simulink model "single_camera_xy_tracking_base_cv_kf"  (R2025b)
settings: Solver=FixedStepDiscrete  StartTime=0  StopTime=T_end  FixedStep=Ts  RelTol=1e-3
InitFcn:
  | config_dir=fullfile(fileparts(get_param(bdroot,'FileName')),'..','config');
  | addpath(config_dir);
  | init_single_camera_xy_tracking_base_cv_kf;
values from neighbouring files (symbols this model uses):
  Kpx = parameters(3)    [build_single_camera_joint_velocity_direct.m]    (also in build_single_camera_joint_velocity_direct1.m)
  Kpy = parameters(4);",  "k_ff=parameters(5)    [build_single_camera_joint_velocity_direct.m]    (also in build_single_camera_joint_velocity_direct1.m)
  Z_hat = parameters(2)    [build_single_camera_joint_velocity_direct.m]    (also in build_single_camera_joint_velocity_direct1.m)
undefined symbols (not defined in the file or in its folder): a_xy_max, controller_enable, data, data_SL_Info, enable_ekf_feedforward, enable_proportional, ff_ramp_time, joint_buffer_capacity, joint_state_timeout_sec, k_ff, measurement_reset_timeout, nis_position_threshold, nis_velocity_threshold, P0, pending_visual_capacity, Q_kf, R_position, R_velocity, required_valid_frames, sync_allow_extrapolation, sync_clock_reset_threshold_sec, sync_max_bracket_span_sec, sync_max_visual_wait_sec, sync_required_for_control, target_timeout_sec, Ts, v_xy_max
libraries: ros2lib x5, robotmaniplib x2
(part 2 of 2)

== matlab function single_camera_xy_tracking_base_cv_kf/Joint State ROS2 Subscriber/Joint Source Timestamp ==
  data: sec input size=1; joint_source_stamp output size=1; nsec input size=1; joint_source_stamp_valid output size=1
function [joint_source_stamp,joint_source_stamp_valid] = fcn(sec,nsec)
%#codegen
% 将 JointState Header 的 sec/nanosec 校验并转换为 ROS 源时间。
joint_source_stamp=0;
joint_source_stamp_valid=0;
sec=double(sec);
nsec=double(nsec);
ok=isfinite(sec)&&sec>=0&&sec==floor(sec)&& ...
    isfinite(nsec)&&nsec>=0&&nsec<1e9&&nsec==floor(nsec);
if ~ok
    return
end
joint_source_stamp=sec+1e-9*nsec;
joint_source_stamp_valid=double(isfinite(joint_source_stamp)&&joint_source_stamp>0);
end

== matlab function single_camera_xy_tracking_base_cv_kf/Visual Joint Time Alignment/Align JointState to Visual Time ==
  data: position_C input size=[2 1]; aligned_position_C output size=[2 1]; relative_velocity_C input size=[2 1]; position_valid input size=1; velocity_valid input size=1; visual_source_stamp input size=1; visual_source_stamp_valid input size=1; visual_message_is_new input size=1; joint_position input size=[7 1]; joint_velocity input size=[7 1]; joint_count input size=1; joint_age input size=1; joint_source_stamp input size=1; joint_source_stamp_valid input size=1; joint_message_is_new input size=1; sim_time input size=1; parameters input size=[8 1]; aligned_relative_velocity_C output size=[2 1]; aligned_q output size=[7 1]; aligned_qdot output size=[7 1]; aligned_visual_stamp output size=1; aligned_joint_stamp_0 output size=1; aligned_joint_stamp_1 output size=1; sync_alpha output size=1; sync_bracket_span output size=1; sync_wait_time output size=1; sync_valid output size=1; aligned_measurement_is_new output size=1; aligned_position_valid output size=1; aligned_velocity_valid output size=1; sync_drop_reason output size=1; joint_buffer_count output size=1; pending_visual_count output size=1; joint_out_of_order_drop_count output size=1; visual_sync_drop_count output size=1; clock_reset_count output size=1; sync_reset_required output size=1
function [aligned_position_C,aligned_relative_velocity_C,aligned_q, ...
    aligned_qdot,aligned_visual_stamp,aligned_joint_stamp_0, ...
    aligned_joint_stamp_1,sync_alpha,sync_bracket_span,sync_wait_time, ...
    sync_valid,aligned_measurement_is_new,aligned_position_valid, ...
    aligned_velocity_valid,sync_drop_reason,joint_buffer_count, ...
    pending_visual_count,joint_out_of_order_drop_count, ...
    visual_sync_drop_count,clock_reset_count,sync_reset_required] = fcn( ...
    position_C,relative_velocity_C,position_valid,velocity_valid, ...
    visual_source_stamp,visual_source_stamp_valid,visual_message_is_new, ...
    joint_position,joint_velocity,joint_count,joint_age, ...
    joint_source_stamp,joint_source_stamp_valid,joint_message_is_new, ...
    sim_time,parameters)
%#codegen
% 缓存 JointState，并在视觉源时刻包围插值关节状态。
[aligned_position_C,aligned_relative_velocity_C,aligned_q, ...
    aligned_qdot,aligned_visual_stamp,aligned_joint_stamp_0, ...
    aligned_joint_stamp_1,sync_alpha,sync_bracket_span,sync_wait_time, ...
    sync_valid_raw,aligned_measurement_is_new_raw,aligned_position_valid_raw, ...
    aligned_velocity_valid_raw,sync_drop_reason,joint_buffer_count, ...
    pending_visual_count,joint_out_of_order_drop_count, ...
    visual_sync_drop_count,clock_reset_count,sync_reset_required_raw]= ...
    joint_visual_time_aligner_step(position_C,relative_velocity_C, ...
    position_valid,velocity_valid,visual_source_stamp, ...
    visual_source_stamp_valid,visual_message_is_new,joint_position, ...
    joint_velocity,joint_count,joint_age,joint_source_stamp, ...
    joint_source_stamp_valid,joint_message_is_new,sim_time, ...
    parameters(1),parameters(2),parameters(3),parameters(4), ...
    parameters(5),parameters(6),parameters(7),parameters(8));
sync_valid=double(sync_valid_raw);
aligned_measurement_is_new=double(aligned_measurement_is_new_raw);
aligned_position_valid=double(aligned_position_valid_raw);
aligned_velocity_valid=double(aligned_velocity_valid_raw);
sync_reset_required=double(sync_reset_required_raw);
end

== matlab function single_camera_xy_tracking_base_cv_kf/Target ROS2 Subscriber/Unpack ==
  data: data input; target_data output size=[8 1]; is_new input size=1; t input size=1; target_count output size=1; target_age output size=1
function [target_data,target_count,target_age] = fcn(data,is_new,t)
%#codegen
% 缓存带图像源时间戳的固定八元素视觉消息。
persistent last_data last_count last_time
if isempty(last_count)
    last_data=zeros(8,1);
    last_count=0;
    last_time=-1e6;
end
if is_new
    n=numel(data);
    last_data=zeros(8,1);
    for k=1:min(n,8)
        last_data(k)=double(data(k));
    end
    last_count=double(n);
    last_time=t;
end
target_data=last_data;
target_count=last_count;
target_age=max(0,t-last_time);
end

== matlab function single_camera_xy_tracking_base_cv_kf/Target Measurement Validation/Validate Timestamped Visual ==
  data: target_data input size=[8 1]; position_valid output size=1; target_count input size=1; target_age input size=1; target_timeout_sec input size=1; velocity_valid output size=1; position_C output size=[2 1]; relative_velocity_C output size=[2 1]; visual_source_stamp output size=1; visual_source_stamp_valid output size=1
function [position_valid,velocity_valid,position_C,relative_velocity_C, ...
    visual_source_stamp,visual_source_stamp_valid] = fcn( ...
    target_data,target_count,target_age,target_timeout_sec)
%#codegen
% 解析并校验带图像源时间戳的八元素视觉消息。
[position_valid_raw,velocity_valid_raw,position_C,relative_velocity_C, ...
    visual_source_stamp,visual_source_stamp_valid_raw]= ...
    parse_target_measurement(target_data,target_count,target_age, ...
    target_timeout_sec);
position_valid=double(position_valid_raw);
velocity_valid=double(velocity_valid_raw);
visual_source_stamp_valid=double(visual_source_stamp_valid_raw);
end

== matlab function single_camera_xy_tracking_base_cv_kf/Joint State ROS2 Subscriber/Unpack ==
  data: position input; joint_position output size=[7 1]; velocity input; is_new input size=1; t input size=1; joint_count output size=1; joint_velocity output size=[7 1]; joint_age output size=1
function [joint_position,joint_count,joint_velocity,joint_age] = fcn(position,velocity,is_new,t)
%#codegen
persistent last_q last_dq last_count last_time
if isempty(last_count), last_q=zeros(7,1); last_dq=zeros(7,1); last_count=0.0; last_time=-1.0e6; end
if is_new
    np=numel(position); nv=numel(velocity); last_q=zeros(7,1); last_dq=zeros(7,1);
    for k=1:min(np,7), last_q(k)=position(k); end
    for k=1:min(nv,7), last_dq(k)=velocity(k); end
    last_count=double(min(np,nv)); last_time=t;
end
joint_position=last_q; joint_count=last_count; joint_velocity=last_dq; joint_age=max(0.0,t-last_time);
end

== matlab function single_camera_xy_tracking_base_cv_kf/Measured Camera Twist in Base/Measured Twist ==
  data: J_camera_base input size=[6 7]; camera_twist_base output size=[6 1]; joint_velocity input size=[7 1]; T_camera2base input size=[4 4]; joint_motion_valid input; joint_geometry_valid input; camera_motion_valid output; T_camera2base_out output size=[4 4]
function [camera_twist_base,camera_motion_valid,T_camera2base_out] = fcn( ...
    J_camera_base,joint_velocity,T_camera2base,joint_motion_valid, ...
    joint_geometry_valid)
%#codegen
% 使用已校验的实测关节速度计算 Base 系相机 Twist。
camera_twist_base=zeros(6,1);
camera_motion_valid=false;
T_camera2base_out=zeros(4,4);

transform_ok=joint_geometry_valid>.5 && ...
    isequal(size(T_camera2base),[4 4]) && all(isfinite(T_camera2base(:)));
if transform_ok
    T_camera2base_out=T_camera2base;
end
if ~(joint_motion_valid>.5 && transform_ok)
    return
end

if isequal(size(J_camera_base),[6 7]) && numel(joint_velocity)==7 && ...
        all(isfinite(J_camera_base(:))) && all(isfinite(joint_velocity(:)))
    twist=J_camera_base*joint_velocity(:);
    if all(isfinite(twist))
        camera_twist_base=twist;
        camera_motion_valid=true;
    end
end
end

== matlab function single_camera_xy_tracking_base_cv_kf/Camera Measurement to Base/Transform Measurement ==
  data: position_C input size=[2 1]; position_B output size=[2 1]; relative_velocity_C input size=[2 1]; T_camera2base input size=[4 4]; camera_twist_base input size=[6 1]; position_valid input; velocity_valid input; camera_motion_valid input; Z_hat input; velocity_B output size=[2 1]; position_valid_out output; velocity_valid_out output
function [position_B,velocity_B,position_valid_out,velocity_valid_out] = fcn( ...
    position_C,relative_velocity_C,T_camera2base,camera_twist_base, ...
    position_valid,velocity_valid,camera_motion_valid,Z_hat)
%#codegen
% 将相机系位置/相对速度转换为 Base 系位置/绝对速度，包含完整角速度补偿。
[position_B,velocity_B,position_valid_out,velocity_valid_out]= ...
    camera_measurement_to_base(position_C,relative_velocity_C,Z_hat, ...
    T_camera2base,camera_twist_base,position_valid,velocity_valid, ...
    camera_motion_valid);
end
